simulink model "FPB"  (Simulink 7.5)
settings: Solver=ode4  StartTime=0.0  StopTime=T  FixedStep=5.0000e-007  RelTol=1e-3
values from neighbouring files (symbols this model uses):
  A = 1.0    (= 1)    [Sinusoides1.m]
  w = 2*pi*f    [RespFreq.m]    (also in Sinusoides1.m = 57315.2163721)
settings Model: Creator=Leonardo  LastModifiedBy=Leo
settings OptimizationCC: InlineInvariantSignals=on  InitFltsAndDblsToZero=on
settings DebuggingCC: SaveWithParameterizedLinksMsg=none  SignalResolutionControl=TryResolveAllWithWarning  MultiTaskDSMMsg=warning  MultiTaskCondExecSysMsg=none  StrictBusMsg=None
settings RTWCC: IncludeERTFirstTime=on
settings GRTTargetCC: TargetFcnLib=ansi_tfl_tmw.mat

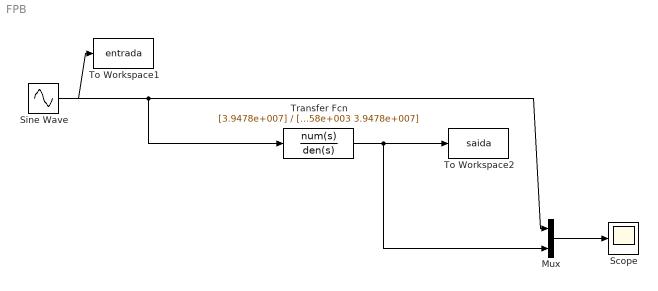
== system FPB ==
  Mux : Mux  Inputs=2
  Scope : Scope
      settings: MaxDataPoints=50000
  Sine Wave : Sin  Amplitude=A  Bias=0  Frequency=w  Phase=0  Samples=10  SampleTime=0  Offset=0
  To Workspace1 : ToWorkspace  VariableName=entrada  SaveFormat=Structure With Time
  To Workspace2 : ToWorkspace  VariableName=saida  SaveFormat=Structure With Time
  Transfer Fcn : TransferFcn  Numerator=[3.9478e+007]  Denominator=[1 8.8858e+003 3.9478e+007]
  wires:
  Mux/1 -> Scope/1
  Transfer Fcn/1 -> To Workspace2/1, Mux/2
  Sine Wave/1 -> Mux/1, To Workspace1/1, Transfer Fcn/1
